simulink model "sensor_wrapper"  (R2020b)
settings: Solver=VariableStepAuto  StartTime=0.0  StopTime=10.0  RelTol=1e-3
settings Model: DataDictionary=sensor_wrapper.sldd  Creator=ravenst1  LastModifiedBy=timoravensbergen

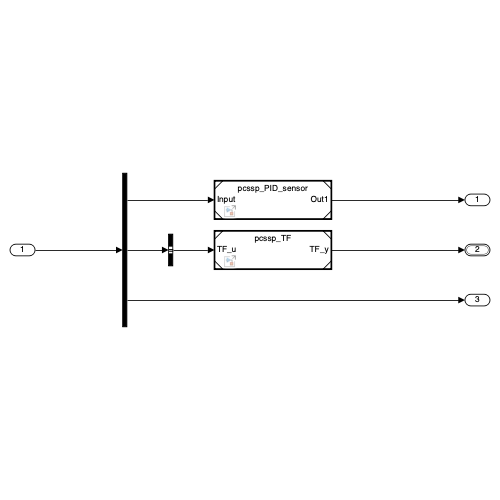
[thumbnail: Simulink's stored preview of the top-level diagram]
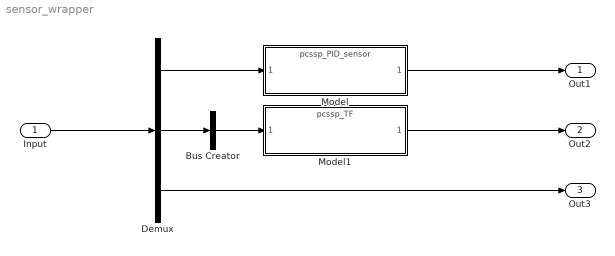
== system sensor_wrapper ==
  Input : Inport
  Bus Creator : BusCreator  Inputs=1  OutDataTypeStr=Bus: pcssp_TF_inBus
      settings: InheritFromInputs=off
  Demux : Demux  Outputs=3
  Model : ModelReference  ModelNameDialog=pcssp_PID_sensor.slx  SimulationMode=Normal  ModelReferenceVersion=1.2
  Model1 : ModelReference  ModelNameDialog=pcssp_TF.slx  SimulationMode=Normal  ModelReferenceVersion=8.1
  Out1 : Outport
  Out2 : Outport  Port=2  OutDataTypeStr=Bus: pcssp_TF_outBus
  Out3 : Outport  Port=3
  wires:
  Model/1 -> Out1/1
  Input/1 -> Demux/1
  Demux/1 -> Model/1
  Model1/1 -> Out2/1
  Demux/3 -> Out3/1
  Bus Creator/1 -> Model1/1
  Demux/2 -> Bus Creator/1
